simulink model "lev"  (R2021b)
settings: Solver=ode3  StartTime=0.0  StopTime=50  FixedStep=1e-4  RelTol=1e-4
values from neighbouring files (symbols this model uses):
  g = 9.8    [MagLev.m]    (also in MagLev4coils.m)
  K = m*g*x1*x1/i/i    (= 2.94e-05)    [MagLev.m]    (also in MagLev4coils.m = m*g*z1*z1/i/i)
  L = 0.00392    [MagLev.m]    (also in MagLev4coils.m = 0.00388)
  m = 0.03    [MagLev.m]    (also in MagLev4coils.m = 0.01)
  R = 4    [MagLev.m]    (also in MagLev4coils.m)
settings Model: Creator=ik76  LastModifiedBy=ik76

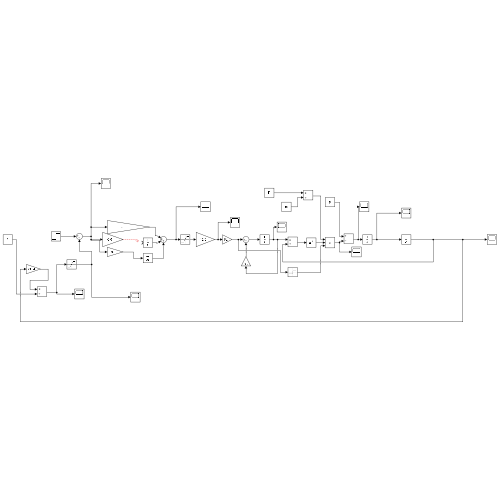
[thumbnail: Simulink's stored preview of the top-level diagram]
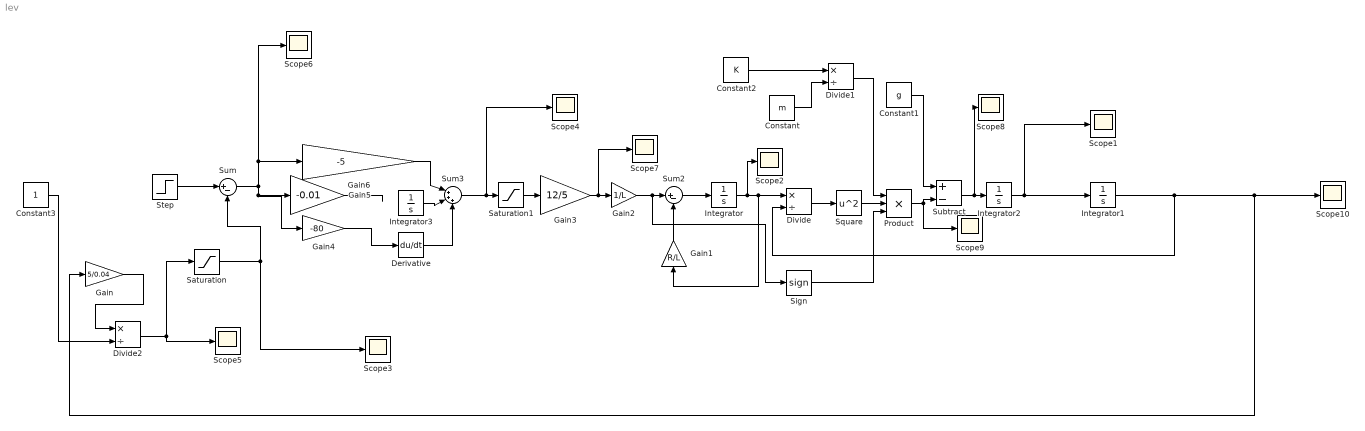
== system lev ==
  Constant : Constant  Value=m
  Constant1 : Constant  Value=g
  Constant2 : Constant  Value=K
  Constant3 : Constant
  Derivative : Derivative
  Divide : Product  Inputs=*/
  Divide1 : Product  Inputs=*/
  Divide2 : Product  Inputs=*/
  Gain : Gain  Gain=5/0.04
  Gain1 : Gain  Gain=R/L
  Gain2 : Gain  Gain=1/L
  Gain3 : Gain  Gain=12/5
  Gain4 : Gain  Gain=-80
  Gain5 : Gain  Gain=-0.01
  Gain6 : Gain  Gain=-5
  Integrator : Integrator
  Integrator1 : Integrator  InitialCondition=0.025
  Integrator2 : Integrator
  Integrator3 : Integrator
  Product : Product  Inputs=3
  Saturation : Saturate  UpperLimit=5  LowerLimit=0
  Saturation1 : Saturate  UpperLimit=5  LowerLimit=-5
  Scope{1..10} (10 alike) : Scope
  Sign : Signum
  Square : Math  Operator=square  SaturateOnIntegerOverflow=on
  Step : Step  Time=0  After=2  SampleTime=0
  Subtract : Sum  Inputs=+-
  Sum : Sum  Inputs=|+-
  Sum2 : Sum  Inputs=|+-
  Sum3 : Sum  Inputs=|+++
  wires:
  Step/1 -> Sum/1
  Gain2/1 -> Sign/1, Sum2/1
  Gain1/1 -> Sum2/2
  Sum2/1 -> Integrator/1
  Integrator/1 -> Scope2/1, Gain1/1, Divide/1
  Divide/1 -> Square/1
  Square/1 -> Product/2
  Product/1 -> Subtract/2, Scope9/1
  Subtract/1 -> Scope8/1, Integrator2/1
  Constant2/1 -> Divide1/1
  Constant/1 -> Divide1/2
  Divide1/1 -> Product/1
  Saturation/1 -> Sum/2, Scope3/1
  Gain3/1 -> Scope7/1, Gain2/1
  Integrator2/1 -> Integrator1/1, Scope1/1
  Gain5/1 -> ?
  Gain4/1 -> Derivative/1
  Gain6/1 -> Sum3/1
  Derivative/1 -> Sum3/3
  Saturation1/1 -> Gain3/1
  Constant1/1 -> Subtract/1
  Sum3/1 -> Saturation1/1, Scope4/1
  Sum/1 -> Gain5/1, Gain4/1, Scope6/1, Gain6/1
  Constant3/1 -> Divide2/2
  Integrator1/1 -> Scope10/1, Gain/1, Divide/2
  Sign/1 -> Product/3
  Divide2/1 -> Saturation/1, Scope5/1
  Gain/1 -> Divide2/1
  Integrator3/1 -> Sum3/2
